simulink model "W1Q2"  (R2020a)
settings: Solver=VariableStepAuto  StartTime=0.0  StopTime=100  RelTol=1e-3
values from neighbouring files (symbols this model uses):
  b = 100    [para.m]
  k1 = 60000    [para.m]
  k2 = 400000    [para.m]
  m1 = 1000    [para.m]
  m2 = 100    [para.m]
settings Model: Creator=Vinayak  LastModifiedBy=Vinayak

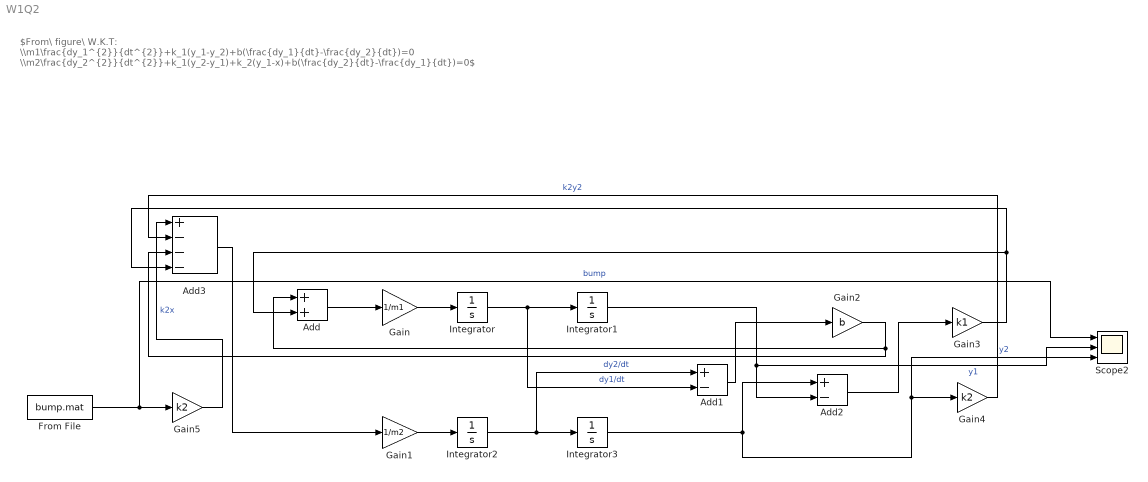
== system W1Q2 ==
  note: $From\ figure\ W.K.T: \\m1\frac{dy_1^{2}}{dt^{2}}+k_1(y_1-y_2)+b(\frac{dy_1}{dt}-\frac{dy_2}{dt})=0 \\m2\frac{dy_2^{2}}{dt^{2}}+k_1(y_2-y_1)+k_2(y_1-x)+b(\frac{dy_2}{dt}-\frac{dy_1}{dt})=0$
  Add : Sum
  Add1 : Sum  Inputs=+-
  Add2 : Sum  Inputs=+-
  Add3 : Sum  Inputs=+---
  From File : FromFile  FileName=bump.mat  SampleTime=0
  Gain : Gain  Gain=1/m1
  Gain1 : Gain  Gain=1/m2
  Gain2 : Gain  Gain=b
  Gain3 : Gain  Gain=k1
  Gain4 : Gain  Gain=k2
  Gain5 : Gain  Gain=k2
  Integrator{,1..3} (4 alike) : Integrator
  Scope2 : Scope  NumInputPorts=3
  wires:
  Gain/1 -> Integrator/1
  Gain1/1 -> Integrator2/1
  Integrator/1 -> Add1/2, Integrator1/1  "dy1/dt"
  Gain4/1 -> Add3/2  "k2y2"
  Integrator2/1 -> Add1/1, Integrator3/1  "dy2/dt"
  Add1/1 -> Gain2/1
  From File/1 -> Scope2/1, Gain5/1  "bump"
  Gain5/1 -> Add3/1  "k2x"
  Gain2/1 -> Add3/3, Add/1
  Gain3/1 -> Add3/4, Add/2
  Add3/1 -> Gain1/1
  Integrator1/1 -> Scope2/2, Add2/2  "y1"
  Add/1 -> Gain/1
  Add2/1 -> Gain3/1
  Integrator3/1 -> Scope2/3, Gain4/1, Add2/1  "y2"
